simulink model "VB_RIFKF_UWB_INS25"  (R2023a)
settings: Solver=FixedStepAuto  StartTime=0.0  StopTime=500  FixedStep=0.01  RelTol=1e-3
InitFcn:
  | resilient_initNavigation1216;
  | init_param;
  | param_bias;
undefined symbols (not defined in the file or in its folder): dt, g0, gam0_rad, ISUS_flag, lp_GPS_sample_time, lp_Lidar_knoise, lp_Lidar_max, lp_Lidar_min, lp_Lidar_sample_time, lp_Lidar_seed, lp_UWB_knoise, lp_UWB_sample_time, lp_UWB_seed, lp_UWB_XY_max, lp_UWB_XY_min, magnitude, p, P0, P0_RIEKF, param, pd0, pe0, phi0_rad, pn0, psi, psi0_rad, state_dim, vd0, ve0, vn0
libraries: simulink_extras x108, simulink x89, dspstat3 x74, sharedtransform x61, matrix_library x11, sharedTrackingLibrary x8, aerolibconvert2 x5, aerolibtransform2 x5, dspfactors x3
(part 21 of 29)

== system VB_RIFKF_UWB_INS25/ISUS_RIEKF3/INS propogation3/Init_PVQ/Horizontal_attitude ==
  note: fai
  note: gamma
  accl_mean_B_m/s_LPF : Inport  PortDimensions=3
  Magn_mean_B_guess_LPF : Inport  Port=2
  Enable : EnablePort
  Add : Sum  Commented=on  Inputs=+-
  Add1 : Sum
  Add2 : Sum
  Asin : Trigonometry  Operator=asin
  Atan2 : Trigonometry  Commented=on  Operator=atan2
  Data Type Conversion : DataTypeConversion  SaturateOnIntegerOverflow=off  RndMeth=Floor
  Deal with zero : Subsystem
  Degrees to Radians : simulink_extras/Transformations/Degrees to Radians  Commented=on
  Degrees to Radians1 : simulink_extras/Transformations/Degrees to Radians
  Demux : Demux  Outputs=3
  Display : Display
  Divide : Product  Inputs=*/  OutDataTypeStr=single
  Gain1 : Gain  Gain=-1
  Gain2 : Gain  Gain=-1
  Magnetic declination : Constant  Commented=on  Value=param.fusion.magDeclDeg  OutDataTypeStr=single
  Magnetic declination1 : Constant  Value=param.control.MagnheadingCorrection  OutDataTypeStr=uint8
  Math Function : Math  Operator=magnitude^2  SignedPower=on
  Mux : Mux  Inputs=3
  Mux1 : Mux  Inputs=3
  Mux3 : Mux  Commented=on  Inputs=3
  Product : Product  Commented=on  Multiplication=Matrix(*)
  Quaternions to Direction Cosine Matrix : sharedtransform/Quaternions to  Direction Cosine Matrix  Commented=on  aMode=aMode
  Radians to Degrees : simulink_extras/Transformations/Radians to Degrees  Commented=on
  Rotation Angles to Quaternions : sharedtransform/Rotation Angles to Quaternions  rotationOrder=ZYX  aMode=aMode
  Rotation Angles to Quaternions1 : sharedtransform/Rotation Angles to Quaternions  Commented=on  rotationOrder=ZYX  aMode=aMode
  Scope : Scope
  Scope1 : Scope
  Selector : Selector  Commented=on  InputPortWidth=3  IndexOptions=Index vector (dialog)  Indices=[2]  OutputSizes=1
  Selector1 : Selector  Commented=on  InputPortWidth=3  IndexOptions=Index vector (dialog)  Indices=[1]  OutputSizes=1
  Sqrt : Sqrt
  Sum of Elements : Sum  Inputs=+
  Switch : Switch  Threshold=0.5  SaturateOnIntegerOverflow=off  InputSameDT=off
  Terminator : Terminator  Commented=on
  Transpose : Math  Commented=on  Operator=transpose  SignedPower=on
  Trigonometric Function1 : Trigonometry  Operator=atan2
  phi0_rad : Constant  Value=phi0_rad  OutDataTypeStr=single
  phi0_rad1 : Constant  Value=gam0_rad  OutDataTypeStr=single
  psi_zero : Constant  Value=psi  OutDataTypeStr=single
  psi_zero1 : Constant  Commented=on  Value=psi  OutDataTypeStr=single
  quat_0 : Outport  PortDimensions=4
  wires:
  Rotation Angles to Quaternions/1 -> Switch/3, Switch/1
  accl_mean_B_m/s_LPF/1 -> Demux/1
  Sqrt/1 -> Deal with zero/1(In1)
  Deal with zero/1(Out1) -> Divide/2
  Trigonometric Function1/1 -> Gain2/1
  Demux/1 -> Divide/1, Mux/2
  Demux/2 -> Mux/1, Trigonometric Function1/1
  Demux/3 -> Gain1/1
  Sum of Elements/1 -> Sqrt/1
  Divide/1 -> Asin/1
  Mux/1 -> Math Function/1
  Math Function/1 -> Sum of Elements/1
  Mux1/1 -> Rotation Angles to Quaternions/1
  psi_zero/1 -> Degrees to Radians1/1
  Add1/1 -> Mux3/2, Mux1/2
  Add2/1 -> Mux3/3, Mux1/3
  Quaternions to Direction Cosine Matrix/1 -> Transpose/1
  Magn_mean_B_guess_LPF/1 -> Product/2
  Product/1 -> Selector/1, Selector1/1  "magNED"
  Selector1/1 -> Atan2/2  "magN"
  Selector/1 -> Atan2/1  "magE"
  Atan2/1 -> Add/2
  Magnetic declination/1 -> Degrees to Radians/1
  Add/1 -> Radians to Degrees/1, Mux3/1  "psi_calbymag"
  Mux3/1 -> Rotation Angles to Quaternions1/1
  Transpose/1 -> Product/1
  Gain1/1 -> Trigonometric Function1/2, Mux/3
  Degrees to Radians1/1 -> Mux1/1
  Degrees to Radians/1 -> Terminator/1
  Magnetic declination1/1 -> Data Type Conversion/1, Switch/2
  Switch/1 -> Scope1/1, quat_0/1
  Data Type Conversion/1 -> Scope/1
  Radians to Degrees/1 -> Display/1
  Asin/1 -> Add1/2
  phi0_rad/1 -> Add1/1
  phi0_rad1/1 -> Add2/1
  Gain2/1 -> Add2/2

== system VB_RIFKF_UWB_INS25/ISUS_RIEKF3/INS propogation3/Init_PVQ/Subsystem ==
  data : Inport
  Buffer : Buffer  N=50  V=49  OutputFrames=off
  Buffer1 : Buffer  N=50  V=49  OutputFrames=off
  Buffer2 : Buffer  N=50  V=49  ic=-g0  OutputFrames=off
  Demux : Demux  Outputs=3
  Mean4 : dspstat3/Mean  run=off  reset_popup=None  directionMode=Entire input  dimension=3  roiEnable=off  roiType=Rectangles  roiPortion=Entire ROI  roiOutput=Individual statistics for each ROI  roiFlag=off  roundingMode=Floor  overflowMode=off  outputDataTypeStr=Inherit: Same as accumulator  outputMin=[]  outputMax=[]  outputLastDataTypeStr=Inherit: Same as accumulator
  Mean5 : dspstat3/Mean  run=off  reset_popup=None  directionMode=Entire input  dimension=3  roiEnable=off  roiType=Rectangles  roiPortion=Entire ROI  roiOutput=Individual statistics for each ROI  roiFlag=off  roundingMode=Floor  overflowMode=off  outputDataTypeStr=Inherit: Same as accumulator  outputMin=[]  outputMax=[]  outputLastDataTypeStr=Inherit: Same as accumulator
  Mean6 : dspstat3/Mean  run=off  reset_popup=None  directionMode=Entire input  dimension=3  roiEnable=off  roiType=Rectangles  roiPortion=Entire ROI  roiOutput=Individual statistics for each ROI  roiFlag=off  roundingMode=Floor  overflowMode=off  outputDataTypeStr=Inherit: Same as accumulator  outputMin=[]  outputMax=[]  outputLastDataTypeStr=Inherit: Same as accumulator
  Scope : Scope  NumInputPorts=2
  Vector Concatenate : Concatenate  NumInputs=3
  mean_data : Outport
  wires:
  Mean6/1 -> Vector Concatenate/3
  Demux/2 -> Buffer1/1
  Buffer/1 -> Mean4/1  "fbx_buff"
  Mean5/1 -> Vector Concatenate/2
  Buffer2/1 -> Mean6/1  "fbz_buff"
  Demux/1 -> Buffer/1
  Buffer1/1 -> Mean5/1  "fby_buff"
  Demux/3 -> Buffer2/1
  Mean4/1 -> Vector Concatenate/1
  Vector Concatenate/1 -> Scope/2, mean_data/1
  data/1 -> Scope/1, Demux/1

== system VB_RIFKF_UWB_INS25/ISUS_RIEKF3/INS propogation3/Init_PVQ/Subsystem1 ==
  data : Inport
  Buffer : Buffer  N=50  V=49  OutputFrames=off
  Buffer1 : Buffer  N=50  V=49  OutputFrames=off
  Buffer2 : Buffer  N=50  V=49  OutputFrames=off
  Demux : Demux  Outputs=3
  Mean4 : dspstat3/Mean  run=off  reset_popup=None  directionMode=Entire input  dimension=3  roiEnable=off  roiType=Rectangles  roiPortion=Entire ROI  roiOutput=Individual statistics for each ROI  roiFlag=off  roundingMode=Floor  overflowMode=off  outputDataTypeStr=Inherit: Same as accumulator  outputMin=[]  outputMax=[]  outputLastDataTypeStr=Inherit: Same as accumulator
  Mean5 : dspstat3/Mean  run=off  reset_popup=None  directionMode=Entire input  dimension=3  roiEnable=off  roiType=Rectangles  roiPortion=Entire ROI  roiOutput=Individual statistics for each ROI  roiFlag=off  roundingMode=Floor  overflowMode=off  outputDataTypeStr=Inherit: Same as accumulator  outputMin=[]  outputMax=[]  outputLastDataTypeStr=Inherit: Same as accumulator
  Mean6 : dspstat3/Mean  run=off  reset_popup=None  directionMode=Entire input  dimension=3  roiEnable=off  roiType=Rectangles  roiPortion=Entire ROI  roiOutput=Individual statistics for each ROI  roiFlag=off  roundingMode=Floor  overflowMode=off  outputDataTypeStr=Inherit: Same as accumulator  outputMin=[]  outputMax=[]  outputLastDataTypeStr=Inherit: Same as accumulator
  Vector Concatenate : Concatenate  NumInputs=3
  mean_data : Outport
  wires:
  data/1 -> Demux/1
  Vector Concatenate/1 -> mean_data/1
  Mean4/1 -> Vector Concatenate/1
  Demux/3 -> Buffer2/1
  Buffer1/1 -> Mean5/1  "fby_buff"
  Demux/1 -> Buffer/1
  Buffer2/1 -> Mean6/1  "fbz_buff"
  Mean5/1 -> Vector Concatenate/2
  Buffer/1 -> Mean4/1  "fbx_buff"
  Demux/2 -> Buffer1/1
  Mean6/1 -> Vector Concatenate/3

== system VB_RIFKF_UWB_INS25/ISUS_RIEKF3/INS propogation3/Init_PVQ/Subsystem2 ==
  Degrees to Radians1 : simulink_extras/Transformations/Degrees to Radians
  Degrees to Radians2 : simulink_extras/Transformations/Degrees to Radians
  Degrees to Radians3 : simulink_extras/Transformations/Degrees to Radians
  Mux : Mux  Inputs=3
  Rotation Angles to Quaternions : sharedtransform/Rotation Angles to Quaternions  rotationOrder=ZYX  aMode=aMode
  phi : Constant  Value=0.11  OutDataTypeStr=single
  psi_zero : Constant  Value=psi  OutDataTypeStr=single
  theta : Constant  Value=1.17  OutDataTypeStr=single
  Quat0 : Outport
  wires:
  Degrees to Radians1/1 -> Mux/1
  Rotation Angles to Quaternions/1 -> Quat0/1
  phi/1 -> Degrees to Radians2/1
  Mux/1 -> Rotation Angles to Quaternions/1
  theta/1 -> Degrees to Radians3/1
  psi_zero/1 -> Degrees to Radians1/1
  Degrees to Radians3/1 -> Mux/2
  Degrees to Radians2/1 -> Mux/3

== system VB_RIFKF_UWB_INS25/ISUS_RIEKF3/INS propogation3/accl bias compensation/error compensation1 ==
  dda : Inport
  QGC_init : Inport  Port=2
  Add3 : Sum
  Delay : Delay  DelayLength=1  InitialCondition=zeros(3,1)  ExternalReset=Level hold
      settings: InputPortMap=u0,r5
  da : Outport
  wires:
  Delay/1 -> Add3/2
  dda/1 -> Add3/1
  QGC_init/1 -> Delay/2
  Add3/1 -> da/1, Delay/1

== system VB_RIFKF_UWB_INS25/ISUS_RIEKF3/INS propogation3/gyro bias compensation/error compensation ==
  ddg : Inport
  Enable : Inport  Port=2
  QGC_init : Inport  Port=3
  Add3 : Sum
  Delay : Delay  DelayLength=1  InitialCondition=zeros(3,1)  ExternalReset=Level hold
      settings: InputPortMap=u0,r5
  If Action Subsystem1 : Subsystem  TreatAsAtomicUnit=on
  If1 : If  IfExpression=u1 == 1  ShowElse=off
  Scope : Scope
  dg : Outport
  wires:
  Enable/1 -> Scope/1, If1/1
  If1/1 -> If Action Subsystem1/Action
  Delay/1 -> Add3/2
  Add3/1 -> Delay/1, dg/1
  ddg/1 -> Add3/1
  QGC_init/1 -> Delay/2

== system VB_RIFKF_UWB_INS25/ISUS_RIEKF3/INS propogation3/vel//pos update/Kinematic Equation ==
  Cbn : Inport
  Ab : Inport  Port=2
  Add : Sum  Inputs=+-
  Add1 : Sum  Inputs=+-
  Constant : Constant  Value=[0 0 -g0]  OutDataTypeStr=single
  Constant1 : Constant  Value=[0 0 -g0]  OutDataTypeStr=single
  Product : Product  Multiplication=Matrix(*)  RndMeth=Zero
  Product1 : Product  Multiplication=Matrix(*)  RndMeth=Zero
  Scope : Scope
  Scope1 : Scope  NumInputPorts=2
  Transpose : Math  Operator=transpose
  An : Outport
  ab_nog : Outport  Port=2
  wires:
  Cbn/1 -> Transpose/1, Product/1
  Add/1 -> An/1, Scope1/2
  Ab/1 -> Product/2, Add1/1, Scope1/1
  Product/1 -> Scope/1, Add/1
  Constant/1 -> Add/2
  Transpose/1 -> Product1/1  "Cnb"
  Constant1/1 -> Product1/2  "gn"
  Product1/1 -> Add1/2  "gb"
  Add1/1 -> ab_nog/1  "ab_nog"

== system VB_RIFKF_UWB_INS25/ISUS_RIEKF3/INS propogation3/vel//pos update/pos update ==
  dtheta : Inport
  vel_k : Inport  Port=2
  dp : Inport  Port=3
  QGC_init : Inport  Port=4
  p0 : Inport  Port=5
  Add1 : Sum
  Delay1 : Delay  DelayLength=1  InitialConditionSource=Input port  ExternalReset=Rising
      settings: InputPortMap=u0,r5,p4
  Gain1 : Gain  Gain=dt
  MATLAB Function : MATLAB Function  TreatAsAtomicUnit=on
  Reshape1 : Reshape  OutputDimensionality=Column vector (2-D)
  p_k : Outport
  wires:
  p0/1 -> Reshape1/1
  QGC_init/1 -> Delay1/2
  Reshape1/1 -> Delay1/3
  Delay1/1 -> Add1/2
  Gain1/1 -> Add1/1
  vel_k/1 -> Gain1/1
  dtheta/1 -> MATLAB Function/1(dtheta)
  dp/1 -> MATLAB Function/2(KFState_dp)
  Add1/1 -> MATLAB Function/3(pos)
  MATLAB Function/1(pos_correct) -> Delay1/1, p_k/1

== system VB_RIFKF_UWB_INS25/ISUS_RIEKF3/INS propogation3/vel//pos update/vel update ==
  dtheta : Inport
  QGC_init : Inport  Port=2
  An : Inport  Port=3
  KFState_dv : Inport  Port=4
  v0 : Inport  Port=5
  Add : Sum
  Delay : Delay  DelayLength=1  InitialConditionSource=Input port  ExternalReset=Rising
      settings: InputPortMap=u0,r5,p4
  Gain : Gain  Gain=dt
  MATLAB Function : MATLAB Function  TreatAsAtomicUnit=on
  Reshape : Reshape  OutputDimensionality=Column vector (2-D)
  vel_k : Outport
  wires:
  QGC_init/1 -> Delay/2
  Reshape/1 -> Delay/3
  An/1 -> Gain/1
  v0/1 -> Reshape/1
  Gain/1 -> Add/1
  Delay/1 -> Add/2
  KFState_dv/1 -> MATLAB Function/2(KFState_dv)
  dtheta/1 -> MATLAB Function/1(dtheta)
  Add/1 -> MATLAB Function/3(vel)
  MATLAB Function/1(vel_correct) -> Delay/1, vel_k/1

== system VB_RIFKF_UWB_INS25/No.1_Sensor_Data_Process/IMU_Data_Process/Bias Eliminate/Subsystem ==
  data : Inport
  Buffer : Buffer  N=50  V=49  OutputFrames=off
  Buffer1 : Buffer  N=50  V=49  OutputFrames=off
  Buffer2 : Buffer  N=50  V=49  OutputFrames=off
  Demux : Demux  Outputs=3
  Mean4 : dspstat3/Mean  run=off  reset_popup=None  directionMode=Entire input  dimension=3  roiEnable=off  roiType=Rectangles  roiPortion=Entire ROI  roiOutput=Individual statistics for each ROI  roiFlag=off  roundingMode=Floor  overflowMode=off  outputDataTypeStr=Inherit: Same as accumulator  outputMin=[]  outputMax=[]  outputLastDataTypeStr=Inherit: Same as accumulator
  Mean5 : dspstat3/Mean  run=off  reset_popup=None  directionMode=Entire input  dimension=3  roiEnable=off  roiType=Rectangles  roiPortion=Entire ROI  roiOutput=Individual statistics for each ROI  roiFlag=off  roundingMode=Floor  overflowMode=off  outputDataTypeStr=Inherit: Same as accumulator  outputMin=[]  outputMax=[]  outputLastDataTypeStr=Inherit: Same as accumulator
  Mean6 : dspstat3/Mean  run=off  reset_popup=None  directionMode=Entire input  dimension=3  roiEnable=off  roiType=Rectangles  roiPortion=Entire ROI  roiOutput=Individual statistics for each ROI  roiFlag=off  roundingMode=Floor  overflowMode=off  outputDataTypeStr=Inherit: Same as accumulator  outputMin=[]  outputMax=[]  outputLastDataTypeStr=Inherit: Same as accumulator
  Scope : Scope  NumInputPorts=2
  Vector Concatenate : Concatenate  NumInputs=3
  mean_data : Outport
  wires:
  data/1 -> Demux/1, Scope/1
  Vector Concatenate/1 -> mean_data/1, Scope/2
  Mean4/1 -> Vector Concatenate/1
  Demux/3 -> Buffer2/1
  Buffer1/1 -> Mean5/1  "fby_buff"
  Demux/1 -> Buffer/1
  Buffer2/1 -> Mean6/1  "fbz_buff"
  Mean5/1 -> Vector Concatenate/2
  Buffer/1 -> Mean4/1  "fbx_buff"
  Demux/2 -> Buffer1/1
  Mean6/1 -> Vector Concatenate/3

== system VB_RIFKF_UWB_INS25/No.1_Sensor_Data_Process1/IMU_Data_Process/Bias Eliminate/Subsystem ==
  data : Inport
  Buffer : Buffer  N=50  V=49  OutputFrames=off
  Buffer1 : Buffer  N=50  V=49  OutputFrames=off
  Buffer2 : Buffer  N=50  V=49  OutputFrames=off
  Demux : Demux  Outputs=3
  Mean4 : dspstat3/Mean  run=off  reset_popup=None  directionMode=Entire input  dimension=3  roiEnable=off  roiType=Rectangles  roiPortion=Entire ROI  roiOutput=Individual statistics for each ROI  roiFlag=off  roundingMode=Floor  overflowMode=off  outputDataTypeStr=Inherit: Same as accumulator  outputMin=[]  outputMax=[]  outputLastDataTypeStr=Inherit: Same as accumulator
  Mean5 : dspstat3/Mean  run=off  reset_popup=None  directionMode=Entire input  dimension=3  roiEnable=off  roiType=Rectangles  roiPortion=Entire ROI  roiOutput=Individual statistics for each ROI  roiFlag=off  roundingMode=Floor  overflowMode=off  outputDataTypeStr=Inherit: Same as accumulator  outputMin=[]  outputMax=[]  outputLastDataTypeStr=Inherit: Same as accumulator
  Mean6 : dspstat3/Mean  run=off  reset_popup=None  directionMode=Entire input  dimension=3  roiEnable=off  roiType=Rectangles  roiPortion=Entire ROI  roiOutput=Individual statistics for each ROI  roiFlag=off  roundingMode=Floor  overflowMode=off  outputDataTypeStr=Inherit: Same as accumulator  outputMin=[]  outputMax=[]  outputLastDataTypeStr=Inherit: Same as accumulator
  Scope : Scope  NumInputPorts=2
  Vector Concatenate : Concatenate  NumInputs=3
  mean_data : Outport
  wires:
  Mean6/1 -> Vector Concatenate/3
  Demux/2 -> Buffer1/1
  Buffer/1 -> Mean4/1  "fbx_buff"
  Mean5/1 -> Vector Concatenate/2
  Buffer2/1 -> Mean6/1  "fbz_buff"
  Demux/1 -> Buffer/1
  Buffer1/1 -> Mean5/1  "fby_buff"
  Demux/3 -> Buffer2/1
  Mean4/1 -> Vector Concatenate/1
  Vector Concatenate/1 -> Scope/2, mean_data/1
  data/1 -> Scope/1, Demux/1

== system VB_RIFKF_UWB_INS25/No.1_Sensor_Data_Process2/IMU_Data_Process/Bias Eliminate/Subsystem ==
  data : Inport
  Buffer : Buffer  N=50  V=49  OutputFrames=off
  Buffer1 : Buffer  N=50  V=49  OutputFrames=off
  Buffer2 : Buffer  N=50  V=49  OutputFrames=off
  Demux : Demux  Outputs=3
  Mean4 : dspstat3/Mean  run=off  reset_popup=None  directionMode=Entire input  dimension=3  roiEnable=off  roiType=Rectangles  roiPortion=Entire ROI  roiOutput=Individual statistics for each ROI  roiFlag=off  roundingMode=Floor  overflowMode=off  outputDataTypeStr=Inherit: Same as accumulator  outputMin=[]  outputMax=[]  outputLastDataTypeStr=Inherit: Same as accumulator
  Mean5 : dspstat3/Mean  run=off  reset_popup=None  directionMode=Entire input  dimension=3  roiEnable=off  roiType=Rectangles  roiPortion=Entire ROI  roiOutput=Individual statistics for each ROI  roiFlag=off  roundingMode=Floor  overflowMode=off  outputDataTypeStr=Inherit: Same as accumulator  outputMin=[]  outputMax=[]  outputLastDataTypeStr=Inherit: Same as accumulator
  Mean6 : dspstat3/Mean  run=off  reset_popup=None  directionMode=Entire input  dimension=3  roiEnable=off  roiType=Rectangles  roiPortion=Entire ROI  roiOutput=Individual statistics for each ROI  roiFlag=off  roundingMode=Floor  overflowMode=off  outputDataTypeStr=Inherit: Same as accumulator  outputMin=[]  outputMax=[]  outputLastDataTypeStr=Inherit: Same as accumulator
  Scope : Scope  NumInputPorts=2
  Vector Concatenate : Concatenate  NumInputs=3
  mean_data : Outport
  wires:
  data/1 -> Demux/1, Scope/1
  Vector Concatenate/1 -> mean_data/1, Scope/2
  Mean4/1 -> Vector Concatenate/1
  Demux/3 -> Buffer2/1
  Buffer1/1 -> Mean5/1  "fby_buff"
  Demux/1 -> Buffer/1
  Buffer2/1 -> Mean6/1  "fbz_buff"
  Mean5/1 -> Vector Concatenate/2
  Buffer/1 -> Mean4/1  "fbx_buff"
  Demux/2 -> Buffer1/1
  Mean6/1 -> Vector Concatenate/3

== system VB_RIFKF_UWB_INS25/No.1_Sensor_Data_Process3/IMU_Data_Process/Bias Eliminate/Subsystem ==
  data : Inport
  Buffer : Buffer  N=50  V=49  OutputFrames=off
  Buffer1 : Buffer  N=50  V=49  OutputFrames=off
  Buffer2 : Buffer  N=50  V=49  OutputFrames=off
  Demux : Demux  Outputs=3
  Mean4 : dspstat3/Mean  run=off  reset_popup=None  directionMode=Entire input  dimension=3  roiEnable=off  roiType=Rectangles  roiPortion=Entire ROI  roiOutput=Individual statistics for each ROI  roiFlag=off  roundingMode=Floor  overflowMode=off  outputDataTypeStr=Inherit: Same as accumulator  outputMin=[]  outputMax=[]  outputLastDataTypeStr=Inherit: Same as accumulator
  Mean5 : dspstat3/Mean  run=off  reset_popup=None  directionMode=Entire input  dimension=3  roiEnable=off  roiType=Rectangles  roiPortion=Entire ROI  roiOutput=Individual statistics for each ROI  roiFlag=off  roundingMode=Floor  overflowMode=off  outputDataTypeStr=Inherit: Same as accumulator  outputMin=[]  outputMax=[]  outputLastDataTypeStr=Inherit: Same as accumulator
  Mean6 : dspstat3/Mean  run=off  reset_popup=None  directionMode=Entire input  dimension=3  roiEnable=off  roiType=Rectangles  roiPortion=Entire ROI  roiOutput=Individual statistics for each ROI  roiFlag=off  roundingMode=Floor  overflowMode=off  outputDataTypeStr=Inherit: Same as accumulator  outputMin=[]  outputMax=[]  outputLastDataTypeStr=Inherit: Same as accumulator
  Scope : Scope  NumInputPorts=2
  Vector Concatenate : Concatenate  NumInputs=3
  mean_data : Outport
  wires:
  Mean6/1 -> Vector Concatenate/3
  Demux/2 -> Buffer1/1
  Buffer/1 -> Mean4/1  "fbx_buff"
  Mean5/1 -> Vector Concatenate/2
  Buffer2/1 -> Mean6/1  "fbz_buff"
  Demux/1 -> Buffer/1
  Buffer1/1 -> Mean5/1  "fby_buff"
  Demux/3 -> Buffer2/1
  Mean4/1 -> Vector Concatenate/1
  Vector Concatenate/1 -> Scope/2, mean_data/1
  data/1 -> Scope/1, Demux/1

== system VB_RIFKF_UWB_INS25/No.1_Sensor_Data_Process4/IMU_Data_Process/Bias Eliminate/Subsystem ==
  data : Inport
  Buffer : Buffer  N=50  V=49  OutputFrames=off
  Buffer1 : Buffer  N=50  V=49  OutputFrames=off
  Buffer2 : Buffer  N=50  V=49  OutputFrames=off
  Demux : Demux  Outputs=3
  Mean4 : dspstat3/Mean  run=off  reset_popup=None  directionMode=Entire input  dimension=3  roiEnable=off  roiType=Rectangles  roiPortion=Entire ROI  roiOutput=Individual statistics for each ROI  roiFlag=off  roundingMode=Floor  overflowMode=off  outputDataTypeStr=Inherit: Same as accumulator  outputMin=[]  outputMax=[]  outputLastDataTypeStr=Inherit: Same as accumulator
  Mean5 : dspstat3/Mean  run=off  reset_popup=None  directionMode=Entire input  dimension=3  roiEnable=off  roiType=Rectangles  roiPortion=Entire ROI  roiOutput=Individual statistics for each ROI  roiFlag=off  roundingMode=Floor  overflowMode=off  outputDataTypeStr=Inherit: Same as accumulator  outputMin=[]  outputMax=[]  outputLastDataTypeStr=Inherit: Same as accumulator
  Mean6 : dspstat3/Mean  run=off  reset_popup=None  directionMode=Entire input  dimension=3  roiEnable=off  roiType=Rectangles  roiPortion=Entire ROI  roiOutput=Individual statistics for each ROI  roiFlag=off  roundingMode=Floor  overflowMode=off  outputDataTypeStr=Inherit: Same as accumulator  outputMin=[]  outputMax=[]  outputLastDataTypeStr=Inherit: Same as accumulator
  Scope : Scope  NumInputPorts=2
  Vector Concatenate : Concatenate  NumInputs=3
  mean_data : Outport
  wires:
  Mean6/1 -> Vector Concatenate/3
  Demux/2 -> Buffer1/1
  Buffer/1 -> Mean4/1  "fbx_buff"
  Mean5/1 -> Vector Concatenate/2
  Buffer2/1 -> Mean6/1  "fbz_buff"
  Demux/1 -> Buffer/1
  Buffer1/1 -> Mean5/1  "fby_buff"
  Demux/3 -> Buffer2/1
  Mean4/1 -> Vector Concatenate/1
  Vector Concatenate/1 -> Scope/2, mean_data/1
  data/1 -> Scope/1, Demux/1

== system VB_RIFKF_UWB_INS25/相对传感器模拟1/Subsystem/laser model/bias & noise z1 ==
  normal : Inport
  Band-Limited White Noise1 : simulink/Sources/Band-Limited White Noise  Cov=[0.1/57.3*0.1/57.3*0.1]  Ts=0.1  seed=[23341]
  Sum1 : Sum  Inputs=|++
  Uniform Random Number : UniformRandomNumber  Minimum=noise_min  Maximum=noise_max  Seed=noise_seed  SampleTime=lp_UWB_sample_time
  noise_k : Gain  Gain=noise_k
  real : Outport
  wires:
  noise_k/1 -> Sum1/2
  Band-Limited White Noise1/1 -> noise_k/1
  normal/1 -> Sum1/1
  Sum1/1 -> real/1

== system VB_RIFKF_UWB_INS25/相对传感器模拟1/Subsystem/laser model/bias & noise z3 ==
  normal : Inport
  Band-Limited White Noise : simulink/Sources/Band-Limited White Noise  Cov=[0.1/57.3*0.1/57.3*0.1]  Ts=0.1  seed=[23341]
  Sum1 : Sum  Inputs=|++
  Uniform Random Number : UniformRandomNumber  Minimum=noise_min  Maximum=noise_max  Seed=noise_seed  SampleTime=lp_UWB_sample_time
  noise_k : Gain  Gain=noise_k
  real : Outport
  wires:
  Sum1/1 -> real/1
  normal/1 -> Sum1/1
  Band-Limited White Noise/1 -> noise_k/1
  noise_k/1 -> Sum1/2

== system VB_RIFKF_UWB_INS25/相对传感器模拟1/Subsystem2/radar model/Subsystem1 ==
  u : Inport
  Scope : Scope  NumInputPorts=2
  Scope1 : Scope
  Subsystem2 : Subsystem
  Switch : Switch  Criteria=u2 > Threshold  SaturateOnIntegerOverflow=off  InputSameDT=off
  厚尾噪声 : MATLAB Function  TreatAsAtomicUnit=on
  y : Outport
  wires:
  Switch/1 -> y/1, Scope/2
  厚尾噪声/1(y) -> Scope/1, Switch/1
  u/1 -> Switch/3, 厚尾噪声/1(u)
  Subsystem2/1(noise_enable) -> Scope1/1

== system VB_RIFKF_UWB_INS25/相对传感器模拟1/Subsystem2/radar model/bias & noise x ==
  normal : Inport
  Band-Limited White Noise : simulink/Sources/Band-Limited White Noise  Cov=[0.1]  Ts=0.1  seed=[23341]
  Scope : Scope  NumInputPorts=2
  Sum1 : Sum  Inputs=|++
  Uniform Random Number : UniformRandomNumber  Minimum=noise_min  Maximum=noise_max  Seed=noise_seed  SampleTime=lp_UWB_sample_time
  noise_k : Gain  Gain=noise_k
  real : Outport
  wires:
  Uniform Random Number/1 -> Scope/2
  Sum1/1 -> real/1
  normal/1 -> Sum1/1
  Band-Limited White Noise/1 -> noise_k/1
  noise_k/1 -> Sum1/2, Scope/1

== system VB_RIFKF_UWB_INS25/相对传感器模拟1/Subsystem2/radar model/bias & noise x1 ==
  normal : Inport
  Band-Limited White Noise : simulink/Sources/Band-Limited White Noise  Cov=[0.1]  Ts=0.1  seed=[23341]
  Sum1 : Sum  Inputs=|++
  Uniform Random Number : UniformRandomNumber  Minimum=noise_min  Maximum=noise_max  Seed=noise_seed  SampleTime=lp_UWB_sample_time
  noise_k : Gain  Gain=noise_k
  real : Outport
  wires:
  noise_k/1 -> Sum1/2
  Band-Limited White Noise/1 -> noise_k/1
  normal/1 -> Sum1/1
  Sum1/1 -> real/1

== system VB_RIFKF_UWB_INS25/相对传感器模拟2/Subsystem/laser model/bias & noise z1 ==
  normal : Inport
  Band-Limited White Noise1 : simulink/Sources/Band-Limited White Noise  Cov=[0.1/57.3*0.1/57.3*0.1]  Ts=0.1  seed=[23341]
  Sum1 : Sum  Inputs=|++
  Uniform Random Number : UniformRandomNumber  Minimum=noise_min  Maximum=noise_max  Seed=noise_seed  SampleTime=lp_UWB_sample_time
  noise_k : Gain  Gain=noise_k
  real : Outport
  wires:
  Sum1/1 -> real/1
  normal/1 -> Sum1/1
  Band-Limited White Noise1/1 -> noise_k/1
  noise_k/1 -> Sum1/2

== system VB_RIFKF_UWB_INS25/相对传感器模拟2/Subsystem/laser model/bias & noise z3 ==
  normal : Inport
  Band-Limited White Noise : simulink/Sources/Band-Limited White Noise  Cov=[0.1/57.3*0.1/57.3*0.1]  Ts=0.1  seed=[23341]
  Sum1 : Sum  Inputs=|++
  Uniform Random Number : UniformRandomNumber  Minimum=noise_min  Maximum=noise_max  Seed=noise_seed  SampleTime=lp_UWB_sample_time
  noise_k : Gain  Gain=noise_k
  real : Outport
  wires:
  noise_k/1 -> Sum1/2
  Band-Limited White Noise/1 -> noise_k/1
  normal/1 -> Sum1/1
  Sum1/1 -> real/1

== system VB_RIFKF_UWB_INS25/相对传感器模拟2/Subsystem2/radar model/Subsystem1 ==
  u : Inport
  Scope : Scope  NumInputPorts=2
  Scope1 : Scope
  Subsystem2 : Subsystem
  Switch : Switch  Criteria=u2 > Threshold  SaturateOnIntegerOverflow=off  InputSameDT=off
  厚尾噪声 : MATLAB Function  TreatAsAtomicUnit=on
  y : Outport
  wires:
  Subsystem2/1(noise_enable) -> Scope1/1
  u/1 -> 厚尾噪声/1(u), Switch/3
  厚尾噪声/1(y) -> Switch/1, Scope/1
  Switch/1 -> Scope/2, y/1

== system VB_RIFKF_UWB_INS25/相对传感器模拟2/Subsystem2/radar model/bias & noise x ==
  normal : Inport
  Band-Limited White Noise : simulink/Sources/Band-Limited White Noise  Cov=[0.1]  Ts=0.1  seed=[23341]
  Scope : Scope  NumInputPorts=2
  Sum1 : Sum  Inputs=|++
  Uniform Random Number : UniformRandomNumber  Minimum=noise_min  Maximum=noise_max  Seed=noise_seed  SampleTime=lp_UWB_sample_time
  noise_k : Gain  Gain=noise_k
  real : Outport
  wires:
  noise_k/1 -> Scope/1, Sum1/2
  Band-Limited White Noise/1 -> noise_k/1
  normal/1 -> Sum1/1
  Sum1/1 -> real/1
  Uniform Random Number/1 -> Scope/2

== system VB_RIFKF_UWB_INS25/相对传感器模拟2/Subsystem2/radar model/bias & noise x1 ==
  normal : Inport
  Band-Limited White Noise : simulink/Sources/Band-Limited White Noise  Cov=[0.1]  Ts=0.1  seed=[23341]
  Sum1 : Sum  Inputs=|++
  Uniform Random Number : UniformRandomNumber  Minimum=noise_min  Maximum=noise_max  Seed=noise_seed  SampleTime=lp_UWB_sample_time
  noise_k : Gain  Gain=noise_k
  real : Outport
  wires:
  Sum1/1 -> real/1
  normal/1 -> Sum1/1
  Band-Limited White Noise/1 -> noise_k/1
  noise_k/1 -> Sum1/2

== system VB_RIFKF_UWB_INS25/相对传感器模拟3/Subsystem/laser model/bias & noise z1 ==
  normal : Inport
  Band-Limited White Noise1 : simulink/Sources/Band-Limited White Noise  Cov=[0.1/57.3*0.1/57.3*0.1]  Ts=0.1  seed=[23341]
  Sum1 : Sum  Inputs=|++
  Uniform Random Number : UniformRandomNumber  Minimum=noise_min  Maximum=noise_max  Seed=noise_seed  SampleTime=lp_UWB_sample_time
  noise_k : Gain  Gain=noise_k
  real : Outport
  wires:
  Sum1/1 -> real/1
  normal/1 -> Sum1/1
  Band-Limited White Noise1/1 -> noise_k/1
  noise_k/1 -> Sum1/2

== system VB_RIFKF_UWB_INS25/相对传感器模拟3/Subsystem/laser model/bias & noise z3 ==
  normal : Inport
  Band-Limited White Noise : simulink/Sources/Band-Limited White Noise  Cov=[0.1/57.3*0.1/57.3*0.1]  Ts=0.1  seed=[23341]
  Sum1 : Sum  Inputs=|++
  Uniform Random Number : UniformRandomNumber  Minimum=noise_min  Maximum=noise_max  Seed=noise_seed  SampleTime=lp_UWB_sample_time
  noise_k : Gain  Gain=noise_k
  real : Outport
  wires:
  noise_k/1 -> Sum1/2
  Band-Limited White Noise/1 -> noise_k/1
  normal/1 -> Sum1/1
  Sum1/1 -> real/1

== system VB_RIFKF_UWB_INS25/相对传感器模拟3/Subsystem2/radar model/Subsystem1 ==
  u : Inport
  Scope : Scope  NumInputPorts=2
  Scope1 : Scope
  Subsystem2 : Subsystem
  Switch : Switch  Criteria=u2 > Threshold  SaturateOnIntegerOverflow=off  InputSameDT=off
  厚尾噪声 : MATLAB Function  TreatAsAtomicUnit=on
  y : Outport
  wires:
  Subsystem2/1(noise_enable) -> Scope1/1
  u/1 -> 厚尾噪声/1(u), Switch/3
  厚尾噪声/1(y) -> Switch/1, Scope/1
  Switch/1 -> Scope/2, y/1

== system VB_RIFKF_UWB_INS25/相对传感器模拟3/Subsystem2/radar model/bias & noise x ==
  normal : Inport
  Band-Limited White Noise : simulink/Sources/Band-Limited White Noise  Cov=[0.1]  Ts=0.1  seed=[23341]
  Scope : Scope  NumInputPorts=2
  Sum1 : Sum  Inputs=|++
  Uniform Random Number : UniformRandomNumber  Minimum=noise_min  Maximum=noise_max  Seed=noise_seed  SampleTime=lp_UWB_sample_time
  noise_k : Gain  Gain=noise_k
  real : Outport
  wires:
  noise_k/1 -> Scope/1, Sum1/2
  Band-Limited White Noise/1 -> noise_k/1
  normal/1 -> Sum1/1
  Sum1/1 -> real/1
  Uniform Random Number/1 -> Scope/2

== system VB_RIFKF_UWB_INS25/相对传感器模拟3/Subsystem2/radar model/bias & noise x1 ==
  normal : Inport
  Band-Limited White Noise : simulink/Sources/Band-Limited White Noise  Cov=[0.1]  Ts=0.1  seed=[23341]
  Sum1 : Sum  Inputs=|++
  Uniform Random Number : UniformRandomNumber  Minimum=noise_min  Maximum=noise_max  Seed=noise_seed  SampleTime=lp_UWB_sample_time
  noise_k : Gain  Gain=noise_k
  real : Outport
  wires:
  Sum1/1 -> real/1
  normal/1 -> Sum1/1
  Band-Limited White Noise/1 -> noise_k/1
  noise_k/1 -> Sum1/2

== system VB_RIFKF_UWB_INS25/相对传感器模拟4/Subsystem/laser model/bias & noise z1 ==
  normal : Inport
  Band-Limited White Noise1 : simulink/Sources/Band-Limited White Noise  Cov=[0.1/57.3*0.1/57.3*0.1]  Ts=0.1  seed=[23341]
  Sum1 : Sum  Inputs=|++
  Uniform Random Number : UniformRandomNumber  Minimum=noise_min  Maximum=noise_max  Seed=noise_seed  SampleTime=lp_UWB_sample_time
  noise_k : Gain  Gain=noise_k
  real : Outport
  wires:
  noise_k/1 -> Sum1/2
  Band-Limited White Noise1/1 -> noise_k/1
  normal/1 -> Sum1/1
  Sum1/1 -> real/1

== system VB_RIFKF_UWB_INS25/相对传感器模拟4/Subsystem/laser model/bias & noise z3 ==
  normal : Inport
  Band-Limited White Noise : simulink/Sources/Band-Limited White Noise  Cov=[0.1/57.3*0.1/57.3*0.1]  Ts=0.1  seed=[23341]
  Sum1 : Sum  Inputs=|++
  Uniform Random Number : UniformRandomNumber  Minimum=noise_min  Maximum=noise_max  Seed=noise_seed  SampleTime=lp_UWB_sample_time
  noise_k : Gain  Gain=noise_k
  real : Outport
  wires:
  Sum1/1 -> real/1
  normal/1 -> Sum1/1
  Band-Limited White Noise/1 -> noise_k/1
  noise_k/1 -> Sum1/2

== system VB_RIFKF_UWB_INS25/相对传感器模拟4/Subsystem2/radar model/Subsystem1 ==
  u : Inport
  Scope : Scope  NumInputPorts=2
  Scope1 : Scope
  Subsystem2 : Subsystem
  Switch : Switch  Criteria=u2 > Threshold  SaturateOnIntegerOverflow=off  InputSameDT=off
  厚尾噪声 : MATLAB Function  TreatAsAtomicUnit=on
  y : Outport
  wires:
  Switch/1 -> y/1, Scope/2
  厚尾噪声/1(y) -> Scope/1, Switch/1
  u/1 -> Switch/3, 厚尾噪声/1(u)
  Subsystem2/1(noise_enable) -> Scope1/1

== system VB_RIFKF_UWB_INS25/相对传感器模拟4/Subsystem2/radar model/bias & noise x ==
  normal : Inport
  Band-Limited White Noise : simulink/Sources/Band-Limited White Noise  Cov=[0.1]  Ts=0.1  seed=[23341]
  Scope : Scope  NumInputPorts=2
  Sum1 : Sum  Inputs=|++
  Uniform Random Number : UniformRandomNumber  Minimum=noise_min  Maximum=noise_max  Seed=noise_seed  SampleTime=lp_UWB_sample_time
  noise_k : Gain  Gain=noise_k
  real : Outport
  wires:
  Uniform Random Number/1 -> Scope/2
  Sum1/1 -> real/1
  normal/1 -> Sum1/1
  Band-Limited White Noise/1 -> noise_k/1
  noise_k/1 -> Sum1/2, Scope/1

== system VB_RIFKF_UWB_INS25/相对传感器模拟4/Subsystem2/radar model/bias & noise x1 ==
  normal : Inport
  Band-Limited White Noise : simulink/Sources/Band-Limited White Noise  Cov=[0.1]  Ts=0.1  seed=[23341]
  Sum1 : Sum  Inputs=|++
  Uniform Random Number : UniformRandomNumber  Minimum=noise_min  Maximum=noise_max  Seed=noise_seed  SampleTime=lp_UWB_sample_time
  noise_k : Gain  Gain=noise_k
  real : Outport
  wires:
  noise_k/1 -> Sum1/2
  Band-Limited White Noise/1 -> noise_k/1
  normal/1 -> Sum1/1
  Sum1/1 -> real/1

== system VB_RIFKF_UWB_INS25/ER EKF M1/Error State Kalman Filter/Extended Kalman Filter1/Correct1/Sk_m_innovation ==
  Pk/k_1 : Inport
  yMeas : Inport  Port=2
  X : Inport  Port=3
  R : Inport  Port=4
  Abs : Abs  Commented=on  SaturateOnIntegerOverflow=off
  Abs1 : Abs  SaturateOnIntegerOverflow=off
  Add : Sum
  Add1 : Sum  Inputs=+-
  Add2 : Sum
  Constant : Constant  Commented=on  Value=8
  Constant1 : Constant  Commented=on  Value=8
  Constant2 : Constant  Commented=on  Value=12
  Constant3 : Constant  Value=eps
  Constant4 : Constant  Commented=on  Value=15
  Constant5 : Constant  Commented=on  Value=8
  Constant6 : Constant  Value=[eye(6),zeros(6,9)]  OutDataTypeStr=single
  Constant7 : Constant  Commented=on  Value=15
  Constant8 : Constant  Commented=on  Value=12
  Constant9 : Constant  Commented=on  Value=25
  Divide : Product  Inputs=*/
  Extract Diagonal1 : matrix_library/Extract Diagonal
  MATLAB Function : MATLAB Function  Commented=on  TreatAsAtomicUnit=on
  Product : Product  Inputs=3  Multiplication=Matrix(*)
  Product1 : Product  Multiplication=Matrix(*)
  Product2 : Product  Commented=on
  Scope : Scope
  Sqrt1 : Sqrt
  Transpose : Math  Operator=transpose
  yMeas1 : InportShadow  Port=2
  measurement innovation : Outport
  wires:
  Product/1 -> Add/1
  Transpose/1 -> Product/3
  R/1 -> Add/2
  Pk/k_1/1 -> Product/2
  yMeas/1 -> Add1/1
  Constant6/1 -> Product1/1, Product/1, Transpose/1
  X/1 -> Product1/2
  Product1/1 -> Add1/2
  Add/1 -> Extract Diagonal1/1  "S"
  Divide/1 -> measurement innovation/1, Abs/1, Scope/1
  MATLAB Function/1(w) -> Product2/1
  Extract Diagonal1/1 -> Abs1/1
  Add1/1 -> Divide/1
  Sqrt1/1 -> Add2/1
  Abs/1 -> MATLAB Function/1(err)
  Abs1/1 -> Sqrt1/1
  Add2/1 -> Divide/2
  Constant3/1 -> Add2/2
  yMeas1/1 -> Product2/2
  Constant1/1 -> MATLAB Function/2(k0)
  Constant4/1 -> MATLAB Function/3(k1)
  Constant/1 -> MATLAB Function/4(zk0)
  Constant2/1 -> MATLAB Function/5(zk1)

== system VB_RIFKF_UWB_INS25/ER EKF M1/Error State Kalman Filter/Extended Kalman Filter1/Predict/If Action Subsystem ==
  Action Port : ActionPort
  Constant : Constant  Value=0
  Data Store Read : DataStoreRead  DataStoreName=x  IndexOptions=Index vector (dialog)  Indices=1  OutputSizes=1
  Data Store Write : DataStoreWrite  DataStoreName=x  IndexOptions=Index vector (dialog)  Indices=1  OutputSizes=1
  Data Store Write1 : DataStoreWrite  DataStoreName=feedback_flag_18dim  IndexOptions=Index vector (dialog)  Indices=1  OutputSizes=1
  Mux : Mux  Inputs=2
  Selector : Selector  InputPortWidth=18  IndexOptions=Index vector (dialog)  Indices=[16 17 18]  OutputSizes=1
  Zero : Constant  Value=zeros(15,1)  OutDataTypeStr=Inherit: Inherit via back propagation
  wires:
  Constant/1 -> Data Store Write1/1
  Data Store Read/1 -> Selector/1
  Zero/1 -> Mux/1
  Selector/1 -> Mux/2
  Mux/1 -> Data Store Write/1

== system VB_RIFKF_UWB_INS25/ER EKF M1/INS propogation/Init_PVQ/Horizontal_attitude/Deal with zero ==
  In1 : Inport
  Add5 : Sum
  Constant1 : Constant  Value=1e-6  OutDataTypeStr=single
  Out1 : Outport
  wires:
  Constant1/1 -> Add5/2
  In1/1 -> Add5/1
  Add5/1 -> Out1/1

== system VB_RIFKF_UWB_INS25/ER EKF M1/INS propogation/Init_PVQ/Horizontal_attitude2/Deal with zero ==
  In1 : Inport
  Add5 : Sum
  Constant1 : Constant  Value=1e-6  OutDataTypeStr=single
  Out1 : Outport
  wires:
  Constant1/1 -> Add5/2
  In1/1 -> Add5/1
  Add5/1 -> Out1/1

== system VB_RIFKF_UWB_INS25/ER EKF M1/INS propogation/gyro bias compensation/error compensation/If Action Subsystem1 ==
  Action Port : ActionPort  ActionPortLabel=if(u1 == 1)
  Constant : Constant
  Data Store Write : DataStoreWrite  DataStoreName=feedback_flag_18dim  IndexOptions=Index vector (dialog)  Indices=1  OutputSizes=1
  wires:
  Constant/1 -> Data Store Write/1

== system VB_RIFKF_UWB_INS25/ISUS_RIEKF M1/Error State Kalman Filter M1/Extended Kalman Filter M1/Predict/If Action Subsystem ==
  Action Port : ActionPort
  Constant : Constant  Value=0
  Data Store Read : DataStoreRead  DataStoreName=x  IndexOptions=Index vector (dialog)  Indices=1  OutputSizes=1
  Data Store Write : DataStoreWrite  DataStoreName=x  IndexOptions=Index vector (dialog)  Indices=1  OutputSizes=1
  Data Store Write1 : DataStoreWrite  DataStoreName=feedback_flag_18dim  IndexOptions=Index vector (dialog)  Indices=1  OutputSizes=1
  Mux : Mux  Inputs=2
  Selector : Selector  InputPortWidth=18  IndexOptions=Index vector (dialog)  Indices=[16 17 18]  OutputSizes=1
  Zero : Constant  Value=zeros(15,1)  OutDataTypeStr=Inherit: Inherit via back propagation
  wires:
  Constant/1 -> Data Store Write1/1
  Data Store Read/1 -> Selector/1
  Zero/1 -> Mux/1
  Selector/1 -> Mux/2
  Mux/1 -> Data Store Write/1

== system VB_RIFKF_UWB_INS25/ISUS_RIEKF M1/Error State Kalman Filter M1/bak/Simulink Function - State Transition Jacobian/Cal Phi1 ==
  Rbn : Inport
  vn : Inport  Port=2
  pn : Inport  Port=3
  Constant : Constant  Value=dt
  MATLAB Function1 : MATLAB Function  TreatAsAtomicUnit=on
  Reshape : Reshape  OutputDimensionality=Column vector (2-D)
  Reshape1 : Reshape  OutputDimensionality=Column vector (2-D)
  Phi : Outport
  wires:
  Reshape1/1 -> MATLAB Function1/2(pn)
  Reshape/1 -> MATLAB Function1/1(vn)
  pn/1 -> Reshape1/1
  vn/1 -> Reshape/1
  Rbn/1 -> MATLAB Function1/3(Rbn)
  MATLAB Function1/1(Phi) -> Phi/1
  Constant/1 -> MATLAB Function1/4(dt)

== system VB_RIFKF_UWB_INS25/ISUS_RIEKF M1/INS propogation/Init_PVQ/Horizontal_attitude/Deal with zero ==
  In1 : Inport
  Add5 : Sum
  Constant1 : Constant  Value=1e-6  OutDataTypeStr=single
  Out1 : Outport
  wires:
  Constant1/1 -> Add5/2
  In1/1 -> Add5/1
  Add5/1 -> Out1/1

== system VB_RIFKF_UWB_INS25/ISUS_RIEKF M1/INS propogation/gyro bias compensation/error compensation/If Action Subsystem1 ==
  Action Port : ActionPort  ActionPortLabel=if(u1 == 1)
  Constant : Constant
  Data Store Write : DataStoreWrite  DataStoreName=feedback_flag_18dim_RIEKF  IndexOptions=Index vector (dialog)  Indices=1  OutputSizes=1
  wires:
  Constant/1 -> Data Store Write/1

== system VB_RIFKF_UWB_INS25/ISUS_RIEKF M2/Error State Kalman Filter M1/Extended Kalman Filter M1/Predict/If Action Subsystem ==
  Action Port : ActionPort
  Constant : Constant  Value=0
  Data Store Read : DataStoreRead  DataStoreName=x  IndexOptions=Index vector (dialog)  Indices=1  OutputSizes=1
  Data Store Write : DataStoreWrite  DataStoreName=x  IndexOptions=Index vector (dialog)  Indices=1  OutputSizes=1
  Data Store Write1 : DataStoreWrite  DataStoreName=feedback_flag_18dim  IndexOptions=Index vector (dialog)  Indices=1  OutputSizes=1
  Mux : Mux  Inputs=2
  Selector : Selector  InputPortWidth=18  IndexOptions=Index vector (dialog)  Indices=[16 17 18]  OutputSizes=1
  Zero : Constant  Value=zeros(15,1)  OutDataTypeStr=Inherit: Inherit via back propagation
  wires:
  Mux/1 -> Data Store Write/1
  Selector/1 -> Mux/2
  Zero/1 -> Mux/1
  Data Store Read/1 -> Selector/1
  Constant/1 -> Data Store Write1/1

== system VB_RIFKF_UWB_INS25/ISUS_RIEKF M2/Error State Kalman Filter M1/bak/Simulink Function - State Transition Jacobian/Cal Phi1 ==
  Rbn : Inport
  vn : Inport  Port=2
  pn : Inport  Port=3
  Constant : Constant  Value=dt
  MATLAB Function1 : MATLAB Function  TreatAsAtomicUnit=on
  Reshape : Reshape  OutputDimensionality=Column vector (2-D)
  Reshape1 : Reshape  OutputDimensionality=Column vector (2-D)
  Phi : Outport
  wires:
  Constant/1 -> MATLAB Function1/4(dt)
  MATLAB Function1/1(Phi) -> Phi/1
  Rbn/1 -> MATLAB Function1/3(Rbn)
  vn/1 -> Reshape/1
  pn/1 -> Reshape1/1
  Reshape/1 -> MATLAB Function1/1(vn)
  Reshape1/1 -> MATLAB Function1/2(pn)

== system VB_RIFKF_UWB_INS25/ISUS_RIEKF M2/Error State Kalman Filter M3/Extended Kalman Filter M1/Predict/If Action Subsystem ==
  Action Port : ActionPort
  Constant : Constant  Value=0
  Data Store Read : DataStoreRead  DataStoreName=x  IndexOptions=Index vector (dialog)  Indices=1  OutputSizes=1
  Data Store Write : DataStoreWrite  DataStoreName=x  IndexOptions=Index vector (dialog)  Indices=1  OutputSizes=1
  Data Store Write1 : DataStoreWrite  DataStoreName=feedback_flag_18dim  IndexOptions=Index vector (dialog)  Indices=1  OutputSizes=1
  Mux : Mux  Inputs=2
  Selector : Selector  InputPortWidth=18  IndexOptions=Index vector (dialog)  Indices=[16 17 18]  OutputSizes=1
  Zero : Constant  Value=zeros(15,1)  OutDataTypeStr=Inherit: Inherit via back propagation
  wires:
  Constant/1 -> Data Store Write1/1
  Data Store Read/1 -> Selector/1
  Zero/1 -> Mux/1
  Selector/1 -> Mux/2
  Mux/1 -> Data Store Write/1

== system VB_RIFKF_UWB_INS25/ISUS_RIEKF M2/Error State Kalman Filter M3/bak/Simulink Function - State Transition Jacobian/Cal Phi1 ==
  Rbn : Inport
  vn : Inport  Port=2
  pn : Inport  Port=3
  Constant : Constant  Value=dt
  MATLAB Function1 : MATLAB Function  TreatAsAtomicUnit=on
  Reshape : Reshape  OutputDimensionality=Column vector (2-D)
  Reshape1 : Reshape  OutputDimensionality=Column vector (2-D)
  Phi : Outport
  wires:
  Reshape1/1 -> MATLAB Function1/2(pn)
  Reshape/1 -> MATLAB Function1/1(vn)
  pn/1 -> Reshape1/1
  vn/1 -> Reshape/1
  Rbn/1 -> MATLAB Function1/3(Rbn)
  MATLAB Function1/1(Phi) -> Phi/1
  Constant/1 -> MATLAB Function1/4(dt)

== system VB_RIFKF_UWB_INS25/ISUS_RIEKF M2/Error State Kalman Filter M4/Extended Kalman Filter M1/Predict/If Action Subsystem ==
  Action Port : ActionPort
  Constant : Constant  Value=0
  Data Store Read : DataStoreRead  DataStoreName=x  IndexOptions=Index vector (dialog)  Indices=1  OutputSizes=1
  Data Store Write : DataStoreWrite  DataStoreName=x  IndexOptions=Index vector (dialog)  Indices=1  OutputSizes=1
  Data Store Write1 : DataStoreWrite  DataStoreName=feedback_flag_18dim  IndexOptions=Index vector (dialog)  Indices=1  OutputSizes=1
  Mux : Mux  Inputs=2
  Selector : Selector  InputPortWidth=18  IndexOptions=Index vector (dialog)  Indices=[16 17 18]  OutputSizes=1
  Zero : Constant  Value=zeros(15,1)  OutDataTypeStr=Inherit: Inherit via back propagation
  wires:
  Mux/1 -> Data Store Write/1
  Selector/1 -> Mux/2
  Zero/1 -> Mux/1
  Data Store Read/1 -> Selector/1
  Constant/1 -> Data Store Write1/1

== system VB_RIFKF_UWB_INS25/ISUS_RIEKF M2/Error State Kalman Filter M4/bak/Simulink Function - State Transition Jacobian/Cal Phi1 ==
  Rbn : Inport
  vn : Inport  Port=2
  pn : Inport  Port=3
  Constant : Constant  Value=dt
  MATLAB Function1 : MATLAB Function  TreatAsAtomicUnit=on
  Reshape : Reshape  OutputDimensionality=Column vector (2-D)
  Reshape1 : Reshape  OutputDimensionality=Column vector (2-D)
  Phi : Outport
  wires:
  Constant/1 -> MATLAB Function1/4(dt)
  MATLAB Function1/1(Phi) -> Phi/1
  Rbn/1 -> MATLAB Function1/3(Rbn)
  vn/1 -> Reshape/1
  pn/1 -> Reshape1/1
  Reshape/1 -> MATLAB Function1/1(vn)
  Reshape1/1 -> MATLAB Function1/2(pn)

== system VB_RIFKF_UWB_INS25/ISUS_RIEKF M2/INS propogation1/Init_PVQ/Horizontal_attitude/Deal with zero ==
  In1 : Inport
  Add5 : Sum
  Constant1 : Constant  Value=1e-6  OutDataTypeStr=single
  Out1 : Outport
  wires:
  Constant1/1 -> Add5/2
  In1/1 -> Add5/1
  Add5/1 -> Out1/1

== system VB_RIFKF_UWB_INS25/ISUS_RIEKF M2/INS propogation1/gyro bias compensation/error compensation/If Action Subsystem1 ==
  Action Port : ActionPort  ActionPortLabel=if(u1 == 1)
  Constant : Constant
  Data Store Write : DataStoreWrite  DataStoreName=feedback_flag_18dim_RIEKF  IndexOptions=Index vector (dialog)  Indices=1  OutputSizes=1
  wires:
  Constant/1 -> Data Store Write/1

== system VB_RIFKF_UWB_INS25/ISUS_RIEKF M2/INS propogation2/Init_PVQ/Horizontal_attitude/Deal with zero ==
  In1 : Inport
  Add5 : Sum
  Constant1 : Constant  Value=1e-6  OutDataTypeStr=single
  Out1 : Outport
  wires:
  Constant1/1 -> Add5/2
  In1/1 -> Add5/1
  Add5/1 -> Out1/1

== system VB_RIFKF_UWB_INS25/ISUS_RIEKF M2/INS propogation2/gyro bias compensation/error compensation/If Action Subsystem1 ==
  Action Port : ActionPort
  Constant : Constant
  Data Store Write : DataStoreWrite  DataStoreName=feedback_flag_18dim_RIEKF  IndexOptions=Index vector (dialog)  Indices=1  OutputSizes=1
  wires:
  Constant/1 -> Data Store Write/1

== system VB_RIFKF_UWB_INS25/ISUS_RIEKF M3/Error State Kalman Filter M1/Extended Kalman Filter M1/Predict/If Action Subsystem ==
  Action Port : ActionPort
  Constant : Constant  Value=0
  Data Store Read : DataStoreRead  DataStoreName=x  IndexOptions=Index vector (dialog)  Indices=1  OutputSizes=1
  Data Store Write : DataStoreWrite  DataStoreName=x  IndexOptions=Index vector (dialog)  Indices=1  OutputSizes=1
  Data Store Write1 : DataStoreWrite  DataStoreName=feedback_flag_18dim  IndexOptions=Index vector (dialog)  Indices=1  OutputSizes=1
  Mux : Mux  Inputs=2
  Selector : Selector  InputPortWidth=18  IndexOptions=Index vector (dialog)  Indices=[16 17 18]  OutputSizes=1
  Zero : Constant  Value=zeros(15,1)  OutDataTypeStr=Inherit: Inherit via back propagation
  wires:
  Constant/1 -> Data Store Write1/1
  Data Store Read/1 -> Selector/1
  Zero/1 -> Mux/1
  Selector/1 -> Mux/2
  Mux/1 -> Data Store Write/1

== system VB_RIFKF_UWB_INS25/ISUS_RIEKF M3/Error State Kalman Filter M1/bak/Simulink Function - State Transition Jacobian/Cal Phi1 ==
  Rbn : Inport
  vn : Inport  Port=2
  pn : Inport  Port=3
  Constant : Constant  Value=dt
  MATLAB Function1 : MATLAB Function  TreatAsAtomicUnit=on
  Reshape : Reshape  OutputDimensionality=Column vector (2-D)
  Reshape1 : Reshape  OutputDimensionality=Column vector (2-D)
  Phi : Outport
  wires:
  Reshape1/1 -> MATLAB Function1/2(pn)
  Reshape/1 -> MATLAB Function1/1(vn)
  pn/1 -> Reshape1/1
  vn/1 -> Reshape/1
  Rbn/1 -> MATLAB Function1/3(Rbn)
  MATLAB Function1/1(Phi) -> Phi/1
  Constant/1 -> MATLAB Function1/4(dt)

== system VB_RIFKF_UWB_INS25/ISUS_RIEKF M3/INS propogation/Init_PVQ/Horizontal_attitude/Deal with zero ==
  In1 : Inport
  Add5 : Sum
  Constant1 : Constant  Value=1e-6  OutDataTypeStr=single
  Out1 : Outport
  wires:
  Constant1/1 -> Add5/2
  In1/1 -> Add5/1
  Add5/1 -> Out1/1

== system VB_RIFKF_UWB_INS25/ISUS_RIEKF M3/INS propogation/gyro bias compensation/error compensation/If Action Subsystem1 ==
  Action Port : ActionPort  ActionPortLabel=if(u1 == 1)
  Constant : Constant
  Data Store Write : DataStoreWrite  DataStoreName=feedback_flag_18dim_RIEKF  IndexOptions=Index vector (dialog)  Indices=1  OutputSizes=1
  wires:
  Constant/1 -> Data Store Write/1

== system VB_RIFKF_UWB_INS25/ISUS_RIEKF3/Error State Kalman Filter M1/Extended Kalman Filter M1/Correct M1/Subsystem2 ==
  Pk_1_ISIU : Inport
  Pk_2 : Inport  Port=2
  Constant : Constant  Value=ISUS_flag
  Data Type Conversion : DataTypeConversion  OutDataTypeStr=single  SaturateOnIntegerOverflow=off  RndMeth=Floor
  MATLAB Function1 : MATLAB Function  TreatAsAtomicUnit=on
  y1 : Outport
  wires:
  Data Type Conversion/1 -> MATLAB Function1/1(u)
  Constant/1 -> MATLAB Function1/3(ISUS_flag)
  Pk_2/1 -> MATLAB Function1/2(X)
  Pk_1_ISIU/1 -> Data Type Conversion/1
  MATLAB Function1/1(y) -> y1/1

== system VB_RIFKF_UWB_INS25/ISUS_RIEKF3/Error State Kalman Filter M1/Extended Kalman Filter M1/Correct M1/innovation calculation ==
  Pk/k_1 : Inport
  yMeas : Inport  Port=2
  X : Inport  Port=3
  R : Inport  Port=4
  H : Inport  Port=5
  Add : Sum
  Add1 : Sum  Inputs=+-
  MATLAB Function : MATLAB Function  TreatAsAtomicUnit=on
  Product : Product  Inputs=3  Multiplication=Matrix(*)
  Product1 : Product  Multiplication=Matrix(*)
  Scope1 : Scope
  Scope2 : Scope
  Scope3 : Scope  NumInputPorts=2
  Selector : Selector  InputPortWidth=6  IndexOptions=Index vector (dialog)  Indices=[4]  OutputSizes=1
  Selector1 : Selector  InputPortWidth=6  IndexOptions=Index vector (dialog)  Indices=[4]  OutputSizes=1
  Transpose : Math  Operator=transpose
  Sk : Outport
  m_innov : Outport  Port=2
  wires:
  Selector1/1 -> Scope3/2
  Selector/1 -> Scope3/1
  Add1/1 -> Scope1/1, m_innov/1, Selector1/1
  Add/1 -> Sk/1  "S"
  Product1/1 -> Add1/2
  X/1 -> Scope2/1, Product1/2
  H/1 -> Transpose/1, Product/1, Product1/1
  yMeas/1 -> Add1/1, Selector/1
  Pk/k_1/1 -> MATLAB Function/1(u)
  R/1 -> Add/2
  Transpose/1 -> Product/3
  Product/1 -> Add/1
  MATLAB Function/1(y) -> Product/2

== system VB_RIFKF_UWB_INS25/ISUS_RIEKF3/Error State Kalman Filter M1/Extended Kalman Filter M1/Predict/If Action Subsystem ==
  Action Port : ActionPort
  Constant : Constant  Value=0
  Data Store Read : DataStoreRead  DataStoreName=x  IndexOptions=Index vector (dialog)  Indices=1  OutputSizes=1
  Data Store Write : DataStoreWrite  DataStoreName=x  IndexOptions=Index vector (dialog)  Indices=1  OutputSizes=1
  Data Store Write1 : DataStoreWrite  DataStoreName=feedback_flag_18dim  IndexOptions=Index vector (dialog)  Indices=1  OutputSizes=1
  Mux : Mux  Inputs=2
  Selector : Selector  InputPortWidth=18  IndexOptions=Index vector (dialog)  Indices=[16 17 18]  OutputSizes=1
  Zero : Constant  Value=zeros(15,1)  OutDataTypeStr=Inherit: Inherit via back propagation
  wires:
  Mux/1 -> Data Store Write/1
  Selector/1 -> Mux/2
  Zero/1 -> Mux/1
  Data Store Read/1 -> Selector/1
  Constant/1 -> Data Store Write1/1
